simulink model "CPG_online"  (R2021b)
settings: Solver=FixedStepDiscrete  StartTime=0.0  StopTime=inf  FixedStep=Ts_cal  MaxStep=0.05  RelTol=0.5  AbsTol=0.5
model workspace (MATLAB code in the model file):
  | %---------------Critical values---------------%
  | angle_amp = pi/4; % Motor rotate amplitude, ref: pi/4
  | rotateCorrectionCoef = 1.158;
  | criticalFn = 2;
  | 
  | %------values for normalization---------------%
  | % values got by running manual gait
  | rotxNormGain = 1/0.1;
  | rotyNormGain = 1/0.05;
  | rotzNormGain = 1/0.1;
  | 
  | vxNormGain = 1/0.2;
  | vyNormGain = 1/0.2;
  | vzNormGain = 1/0.2;
  | 
  | FnNormGain = 1/15;
  | 
  | %--------values for check done---------------%
  | rotDone = pi/6;
  | legBendDone = pi/3; % actuator max bending angle
  | 
  | %---------------Robot parameters-------------%
  | % robot size
  | robot_width = 0.15;
  | robot_length = 0.22;
  | 
  | % floor parameters
  | floor_length = 2;
  | floor_width = 2;
  | 
  | % continuum actuator size
  | L_disk = 0.02944;% Disk side length (m)
  | R_w = L_disk/sqrt(3);
  | thickness_disk = 0.004; % Disk thickness (m)
  | thigh_length = 0.06;
  | R_core = 0.005; % Core radius (m)
  | length_core = 0.008; % Core length (m)
  | R_spool = 0.021; % 0.01944; % radius of the spool
  | spool_height = 0.022+0.015;
  | R_pulley = 1e-3;
  | spool_k = 0;
  | spool_d = 0;
  | hole_d = 4e-3;
  | 
  | % Material property
  | rho_PLA = 1.24e3;
  | rho = 1.19e3; % 1.19e3; % Density (kg/m^3)
  | % use rigid joints
  | Pz_stiff = 135000;
  | Pz_damping = 500;
  | S_stiff = 0.0239;
  | S_damping = 7.5e-5;
  | S_low_Bound = -20;
  | S_up_Bound = 20;
  | 
  | R_foot = 0.015; % foot radius (m)
  | 
  | % motor parameter
  | stall_T = 11.2/10; % 11.2 cm*kg, stall torque
  | t_60_deg = 0.2; % 0.09 s
  | V_nomrmal = 6; % corresponding normal voltage
  | Jr = 0.0001; %g*cm^2, robot inertia
  | 
  | % contact force
  | coef_static_friction = 0.315;
  | coef_dynamic_friction = 0.3;
  | crictic_velocity = 0.3; % m/s
  | contact_suf_stiff = 1000; % N/m
  | contact_suf_damp = 50; % N/(m/s)
  | contact_region_width = 2e-3; % m
  | spoolOpacity = 0;
  | tendonColor = [0.902 0.902 0.902];
  | tendonOpacity = 0.1;
  | 
  | % If use point masses
  | MMainFrame = 198; % g
  | MServoMotor = 50.55;
  | MMotorSupport = 12.1;
  | MSpool = 9.2;
  | 
  | % Robot total weight about 2 kg
  | MComposateLoad = 200;
  | 
  | MBuck = 40; % x2
  | MPCB_RPi = 141.3;
  | MLiBattery = 120; % x2
  | MPowerBank = 66.5;
  | isLoadVisible = 0.1;
  | 
  | 
  | MThigh = 26.7963;
  | MCore = 0.747699;
  | MDisk = 1.78642;
  | MFoot = 16.8232;
values from neighbouring files (symbols this model uses):
  A = [0 Ts; 0 1]    [MFBO_main.m]    (also in MFGP_main.m)
  A_cpg = 1    [MFBO_main.m]    (also in MFGP_main.m)
  alpha = opt_param(2)    [MFBO_main.m]    (also in MFGP_main.m)
  alpha_b_gain = opt_param(3)    [MFBO_main.m]    (also in MFGP_main.m)
  alpha_r_gain = pi    (= 3.14159265359)    [MFBO_main.m]    (also in MFGP_main.m)
  B = [0.5*Ts^2; Ts]    [MFBO_main.m]    (also in MFGP_main.m)
  C = [1 0]    [MFBO_main.m]    (also in MFGP_main.m)
  epsilon = 5    [MFBO_main.m]    (also in MFGP_main.m)
  f = 1/T    [MFBO_main.m]    (also in MFGP_main.m)
  init_state = rand(1, 8)*2 - 1    [MFBO_main.m]    (also in MFGP_main.m)
  k = 1000    [MFBO_main.m]    (also in MFGP_main.m)
  phi_vec = pi*[-1; 1; -1; 1]    [MFBO_main.m]    (also in MFGP_main.m)
  R = 0.15    [MFBO_main.m]    (also in MFGP_main.m)
  tau = 1    [MFBO_main.m]    (also in MFGP_main.m)
  Ts = 5e-2    (= 0.05)    [MFBO_main.m]    (also in MFGP_main.m)
  Ts_cal = 5e-4    (= 0.0005)    [MFBO_main.m]    (also in MFGP_main.m)
  z_l_diff = opt_param(5)    [MFBO_main.m]    (also in MFGP_main.m)
  z_l_gain = opt_param(4)    [MFBO_main.m]    (also in MFGP_main.m)
undefined symbols (not defined in the file or in its folder): DiscIntNeverNeededParam, Discrete, Time
libraries: svdutilitieslib x15, simulink x4, ctrlSharedLib x3, instrumentlib x2, aerolibanimutils x1
(part 2 of 2)

== system CPG_online/Sensing/vy_cal ==
  left : Inport
  right : Inport  Port=2
  acc_y : Inport  Port=3
  Add : Sum  Inputs=+-
  Add1 : Sum  Inputs=+-
  Data Type Conversion1 : DataTypeConversion  OutDataTypeStr=double
  Data Type Conversion10 : DataTypeConversion  OutDataTypeStr=double
  Data Type Conversion9 : DataTypeConversion  OutDataTypeStr=double
  Delay : Delay  SampleTime=Ts
  Delay1 : Delay  DelayLength=1  SampleTime=Ts
  Delay2 : Delay  DelayLength=1  SampleTime=Ts
  Delay3 : Delay  DelayLength=1  SampleTime=Ts
  Gain : Gain  Gain=1/1000
  Gain12 : Gain  Gain=-1
  Kalman Filter : ctrlSharedLib/Kalman Filter  TimeDomain=Discrete-Time  UseCurrentEstimator=on  ModelSource=Individual A, B, C, D matrices  ModelSourceVariable=ss(0.95,1,1,0,1)  A=A  B=B  C=C  D=0  NumberOfStates=1  NumberOfInputs=1  NumberOfOutputs=1  InitialEstimateSource=Dialog  X0=[0;0]  P0=10  UseK=off  UseGH=off  NumberOfProcessNoiseInputs=1  G=1  TimeInvariantG=on  H=0  TimeInvariantH=on  Q=Q  TimeInvariantQ=on  R=R  TimeInvariantR=on  N=0  TimeInvariantN=on  AddInputPort=on  AddEnablePort=off  OutputEstimatedY=off  OutputP=off  Ts=Ts
  MATLAB Function : MATLAB Function  TreatAsAtomicUnit=on
  MATLAB Function1 : MATLAB Function  TreatAsAtomicUnit=on
  MATLAB Function2 : MATLAB Function  TreatAsAtomicUnit=on
  Terminator : Terminator
  vy : Outport
  wires:
  Delay1/1 -> MATLAB Function1/3(predd_acc)
  Delay/1 -> MATLAB Function1/2(pred_acc), Delay1/1
  acc_y/1 -> Data Type Conversion1/1
  MATLAB Function1/1(acceleration) -> Kalman Filter/1  "acc"
  Delay3/1 -> Add1/2
  Gain12/1 -> MATLAB Function/1(v_left)
  Data Type Conversion10/1 -> Delay2/1, Add/1  "v_left"
  right/1 -> Data Type Conversion10/1
  MATLAB Function/1(vy) -> Gain/1  "vy"
  left/1 -> Data Type Conversion9/1
  Data Type Conversion9/1 -> Add1/1, Delay3/1  "v_left"
  Gain/1 -> Kalman Filter/2  "vy"
  Delay2/1 -> Add/2
  Add/1 -> MATLAB Function/2(v_right)
  Add1/1 -> Gain12/1
  Data Type Conversion1/1 -> Delay/1, MATLAB Function1/1("acceleration ")
  Kalman Filter/1 -> MATLAB Function2/1(u)  "vy"
  MATLAB Function2/1(y) -> Terminator/1
  MATLAB Function2/2(v) -> vy/1

== system CPG_online/Sensing/vz_cal ==
  down : Inport
  acc_z : Inport  Port=2
  Add1 : Sum  Inputs=+-
  Data Type Conversion1 : DataTypeConversion  OutDataTypeStr=double
  Data Type Conversion9 : DataTypeConversion  OutDataTypeStr=double
  Delay : Delay  SampleTime=Ts
  Delay1 : Delay  DelayLength=1  SampleTime=Ts
  Delay3 : Delay  DelayLength=1  SampleTime=Ts
  Gain : Gain  Gain=1/1000
  Gain12 : Gain  Gain=-1
  Kalman Filter : ctrlSharedLib/Kalman Filter  TimeDomain=Discrete-Time  UseCurrentEstimator=on  ModelSource=Individual A, B, C, D matrices  ModelSourceVariable=ss(0.95,1,1,0,1)  A=A  B=B  C=C  D=0  NumberOfStates=1  NumberOfInputs=1  NumberOfOutputs=1  InitialEstimateSource=Dialog  X0=[0;0]  P0=10  UseK=off  UseGH=off  NumberOfProcessNoiseInputs=1  G=1  TimeInvariantG=on  H=0  TimeInvariantH=on  Q=Q  TimeInvariantQ=on  R=R  TimeInvariantR=on  N=0  TimeInvariantN=on  AddInputPort=on  AddEnablePort=off  OutputEstimatedY=off  OutputP=off  Ts=Ts
  MATLAB Function : MATLAB Function  TreatAsAtomicUnit=on
  MATLAB Function1 : MATLAB Function  TreatAsAtomicUnit=on
  MATLAB Function2 : MATLAB Function  TreatAsAtomicUnit=on
  Terminator : Terminator
  vz : Outport
  wires:
  Delay1/1 -> MATLAB Function1/3(predd_acc)
  Delay/1 -> MATLAB Function1/2(pred_acc), Delay1/1
  acc_z/1 -> Data Type Conversion1/1
  MATLAB Function1/1(acceleration) -> Kalman Filter/1  "acc"
  Delay3/1 -> Add1/2
  Gain12/1 -> MATLAB Function/1(v_down)
  MATLAB Function/1(vz) -> Gain/1  "vz"
  down/1 -> Data Type Conversion9/1
  Data Type Conversion9/1 -> Add1/1, Delay3/1
  Gain/1 -> Kalman Filter/2  "vz"
  Add1/1 -> Gain12/1  "v_down"
  Data Type Conversion1/1 -> Delay/1, MATLAB Function1/1("acceleration ")
  Kalman Filter/1 -> MATLAB Function2/1(u)  "vz"
  MATLAB Function2/2(v) -> vz/1
  MATLAB Function2/1(y) -> Terminator/1

== system CPG_online/Subsystem/FL ==
  act : Inport
  Add : Sum
  Constant : Constant
  Demux1 : Demux  Outputs=3
  Gain : Gain  Gain=alpha_r_gain
  Gain1 : Gain  Gain=alpha_b_gain
  Gain2 : Gain  Gain=z_l_gain/2
  MATLAB Function : MATLAB Function  TreatAsAtomicUnit=on
  Mux3 : Mux  Inputs=3
  angle : Outport
  wires:
  MATLAB Function/3(alpha_C) -> Mux3/3
  Demux1/2 -> Gain1/1  "alpha_b_Ref"
  Gain1/1 -> MATLAB Function/2(alpha_b)
  Constant/1 -> Add/2
  MATLAB Function/1(alpha_A) -> Mux3/1
  MATLAB Function/2(alpha_B) -> Mux3/2
  Gain2/1 -> MATLAB Function/3(z_l)
  Demux1/3 -> Add/1  "z_l_Ref"
  Demux1/1 -> Gain/1  "alpha_r_Ref"
  Gain/1 -> MATLAB Function/1(alpha_r)
  Add/1 -> Gain2/1
  Mux3/1 -> angle/1
  act/1 -> Demux1/1

== system CPG_online/Subsystem/FR ==
  act : Inport
  Add : Sum
  Constant : Constant
  Demux1 : Demux  Outputs=3
  Gain : Gain  Gain=alpha_r_gain
  Gain1 : Gain  Gain=alpha_b_gain
  Gain2 : Gain  Gain=z_l_gain/2
  MATLAB Function : MATLAB Function  TreatAsAtomicUnit=on
  Mux3 : Mux  Inputs=3
  angle : Outport
  wires:
  MATLAB Function/3(alpha_C) -> Mux3/3
  Demux1/2 -> Gain1/1  "alpha_b_Ref"
  Gain1/1 -> MATLAB Function/2(alpha_b)
  Constant/1 -> Add/2
  MATLAB Function/1(alpha_A) -> Mux3/1
  MATLAB Function/2(alpha_B) -> Mux3/2
  Gain2/1 -> MATLAB Function/3(z_l)
  Demux1/3 -> Add/1  "z_l_Ref"
  Demux1/1 -> Gain/1  "alpha_r_Ref"
  Gain/1 -> MATLAB Function/1(alpha_r)
  Add/1 -> Gain2/1
  Mux3/1 -> angle/1
  act/1 -> Demux1/1

== system CPG_online/Subsystem/RL ==
  act : Inport
  Add : Sum
  Constant : Constant
  Demux1 : Demux  Outputs=3
  Gain : Gain  Gain=alpha_r_gain
  Gain1 : Gain  Gain=alpha_b_gain
  Gain2 : Gain  Gain=z_l_gain/2
  MATLAB Function : MATLAB Function  TreatAsAtomicUnit=on
  Mux3 : Mux  Inputs=3
  angle : Outport
  wires:
  MATLAB Function/3(alpha_C) -> Mux3/3
  Demux1/2 -> Gain1/1  "alpha_b_Ref"
  Gain1/1 -> MATLAB Function/2(alpha_b)
  Constant/1 -> Add/2
  MATLAB Function/1(alpha_A) -> Mux3/1
  MATLAB Function/2(alpha_B) -> Mux3/2
  Gain2/1 -> MATLAB Function/3(z_l)
  Demux1/3 -> Add/1  "z_l_Ref"
  Demux1/1 -> Gain/1  "alpha_r_Ref"
  Gain/1 -> MATLAB Function/1(alpha_r)
  Add/1 -> Gain2/1
  Mux3/1 -> angle/1
  act/1 -> Demux1/1

== system CPG_online/Subsystem/RR ==
  act : Inport
  Add : Sum
  Constant : Constant
  Demux1 : Demux  Outputs=3
  Gain : Gain  Gain=alpha_r_gain
  Gain1 : Gain  Gain=alpha_b_gain
  Gain2 : Gain  Gain=z_l_gain/2
  MATLAB Function : MATLAB Function  TreatAsAtomicUnit=on
  Mux3 : Mux  Inputs=3
  angle : Outport
  wires:
  MATLAB Function/3(alpha_C) -> Mux3/3
  Demux1/2 -> Gain1/1  "alpha_b_Ref"
  Gain1/1 -> MATLAB Function/2(alpha_b)
  Constant/1 -> Add/2
  MATLAB Function/1(alpha_A) -> Mux3/1
  MATLAB Function/2(alpha_B) -> Mux3/2
  Gain2/1 -> MATLAB Function/3(z_l)
  Demux1/3 -> Add/1  "z_l_Ref"
  Demux1/1 -> Gain/1  "alpha_r_Ref"
  Gain/1 -> MATLAB Function/1(alpha_r)
  Add/1 -> Gain2/1
  Mux3/1 -> angle/1
  act/1 -> Demux1/1

== system CPG_online/Sensing/rot_cal/Subsystem ==
  rotz_raw : Inport
  Abs : Abs
  Delay : Delay  DelayLength=1
  Subtract : Sum  Inputs=-+
  Switch : Switch  Criteria=u2 > Threshold  Threshold=0.2
  rotz : Outport
  wires:
  rotz_raw/1 -> Switch/3, Subtract/2
  Delay/1 -> Switch/1, Subtract/1
  Abs/1 -> Switch/2
  Subtract/1 -> Abs/1
  Switch/1 -> Delay/1, rotz/1

== system CPG_online/Sensing/rot_cal/Subsystem1 ==
  roty_raw : Inport
  Abs : Abs
  Delay : Delay  DelayLength=1
  Subtract : Sum  Inputs=-+
  Switch : Switch  Criteria=u2 > Threshold  Threshold=0.2
  roty : Outport
  wires:
  roty_raw/1 -> Switch/3, Subtract/2
  Delay/1 -> Switch/1, Subtract/1
  Abs/1 -> Switch/2
  Subtract/1 -> Abs/1
  Switch/1 -> Delay/1, roty/1

== system CPG_online/Sensing/rot_cal/Subsystem2 ==
  rotx_raw : Inport
  Abs : Abs
  Delay : Delay  DelayLength=1
  Subtract : Sum  Inputs=-+
  Switch : Switch  Criteria=u2 > Threshold  Threshold=0.2
  rotx : Outport
  wires:
  rotx_raw/1 -> Switch/3, Subtract/2
  Delay/1 -> Switch/1, Subtract/1
  Abs/1 -> Switch/2
  Subtract/1 -> Abs/1
  Switch/1 -> Delay/1, rotx/1

== matlab function CPG_online/Subsystem/RL/MATLAB Function ==
  data: alpha_r input; alpha_A output; alpha_b input; z_l input; alpha_B output; alpha_C output
function [alpha_A, alpha_B, alpha_C]= fcn(alpha_r, alpha_b, z_l)

L_disk = 0.02944;% Disk side length (m)
R_spool = 0.021;
R_w = L_disk/sqrt(3);

alpha_A = (-R_w*alpha_b*cos(-alpha_r)+z_l)/R_spool;
alpha_B = (-R_w*alpha_b*cos(-alpha_r+2*pi/3)+z_l)/R_spool;
alpha_C = (-R_w*alpha_b*cos(-alpha_r+4*pi/3)+z_l)/R_spool;

== matlab function CPG_online/CPG_cont/Hopf_oscillator (leg#2)/adaptive_f ==
  data: alpha input; f_a output; f input; tau input; v input
 % calculate the adaptive frequency f through (4) in 
 % 'Design and Locomotion Control of a Biomimetic Underwater Vehicle ... '
function f_a = adaptive_f(alpha, f, tau, v)
    f1 = f/2/alpha;
    f2 = (2*alpha - 1)*f/(2*alpha*(1 - alpha)*(1 + exp(-tau*v)));
    f_a = f1 + f2;

== matlab function CPG_online/CPG_cont/Hopf_oscillator (leg#3)/adaptive_f ==
  data: alpha input; f_a output; f input; tau input; v input
 % calculate the adaptive frequency f through (4) in 
 % 'Design and Locomotion Control of a Biomimetic Underwater Vehicle ... '
function f_a = adaptive_f(alpha, f, tau, v)
    f1 = f/2/alpha;
    f2 = (2*alpha - 1)*f/(2*alpha*(1 - alpha)*(1 + exp(-tau*v)));
    f_a = f1 + f2;

== matlab function CPG_online/Sensing/vy_cal/MATLAB Function ==
  data: v_left input; vy output; v_right input
function vy = fcn(v_left, v_right)

if abs(v_left) >= 20 && abs(v_right) < 20
    vy = v_right;
elseif abs(v_right) >= 20 && abs(v_left) < 20
    vy = v_left;
else
    vy = (v_right + v_left)/2;
end

== matlab function CPG_online/CPG_cont/Hopf_oscillator (leg#4)/adaptive_f ==
  data: alpha input; f_a output; f input; tau input; v input
 % calculate the adaptive frequency f through (4) in 
 % 'Design and Locomotion Control of a Biomimetic Underwater Vehicle ... '
function f_a = adaptive_f(alpha, f, tau, v)
    f1 = f/2/alpha;
    f2 = (2*alpha - 1)*f/(2*alpha*(1 - alpha)*(1 + exp(-tau*v)));
    f_a = f1 + f2;

== matlab function CPG_online/CPG_cont/leg_coupling ==
  data: epsilon input; u_vec input; C_leg1 output size=2; v_vec input; phi_vec input; C_leg2 output size=2; C_leg3 output size=2; C_leg4 output size=2
% epsilon: 1X1
% u_vec: 4X1
% v_vec: 4X1
% phi_vec: 4X1
% C_leg1-4 : 2X1
function [C_leg1, C_leg2, C_leg3, C_leg4] = fcn(epsilon, u_vec, v_vec, phi_vec)
    C1 = 0;
    % first leg
    C21 = epsilon*(-u_vec(4)*sin(phi_vec(4)) + v_vec(4)*cos(phi_vec(4)) - ...
                   -u_vec(1)*sin(phi_vec(1)) + v_vec(2)*cos(phi_vec(1)));
    C22 = epsilon*(-u_vec(1)*sin(phi_vec(1)) + v_vec(1)*cos(phi_vec(1)) - ...
                   -u_vec(2)*sin(phi_vec(2)) + v_vec(3)*cos(phi_vec(2)));
    C23 = epsilon*(-u_vec(2)*sin(phi_vec(2)) + v_vec(2)*cos(phi_vec(2)) - ...
                   -u_vec(3)*sin(phi_vec(3)) + v_vec(4)*cos(phi_vec(3)));
    C24 = epsilon*(-u_vec(3)*sin(phi_vec(3)) + v_vec(3)*cos(phi_vec(3)) - ...
                   -u_vec(4)*sin(phi_vec(4)) + v_vec(1)*cos(phi_vec(4)));
    
    C_leg1 = [C1; C21];
    C_leg2 = [C1; C22];
    C_leg3 = [C1; C23];
    C_leg4 = [C1; C24];

== matlab function CPG_online/CPG/Hopf_oscillator (leg#4)/adaptive_f ==
  data: alpha input; f_a output; f input; tau input; v input
 % calculate the adaptive frequency f through (4) in 
 % 'Design and Locomotion Control of a Biomimetic Underwater Vehicle ... '
function f_a = adaptive_f(alpha, f, tau, v)
    f1 = f/2/alpha;
    f2 = (2*alpha - 1)*f/(2*alpha*(1 - alpha)*(1 + exp(-tau*v)));
    f_a = f1 + f2;

== matlab function CPG_online/CPG/leg_coupling ==
  data: epsilon input; u_vec input; C_leg1 output size=2; v_vec input; phi_vec input; C_leg2 output size=2; C_leg3 output size=2; C_leg4 output size=2
% epsilon: 1X1
% u_vec: 4X1
% v_vec: 4X1
% phi_vec: 4X1
% C_leg1-4 : 2X1
function [C_leg1, C_leg2, C_leg3, C_leg4] = fcn(epsilon, u_vec, v_vec, phi_vec)
    C1 = 0;
    % first leg
    C21 = epsilon*(-u_vec(4)*sin(phi_vec(4)) + v_vec(4)*cos(phi_vec(4)) - ...
                   -u_vec(1)*sin(phi_vec(1)) + v_vec(2)*cos(phi_vec(1)));
    C22 = epsilon*(-u_vec(1)*sin(phi_vec(1)) + v_vec(1)*cos(phi_vec(1)) - ...
                   -u_vec(2)*sin(phi_vec(2)) + v_vec(3)*cos(phi_vec(2)));
    C23 = epsilon*(-u_vec(2)*sin(phi_vec(2)) + v_vec(2)*cos(phi_vec(2)) - ...
                   -u_vec(3)*sin(phi_vec(3)) + v_vec(4)*cos(phi_vec(3)));
    C24 = epsilon*(-u_vec(3)*sin(phi_vec(3)) + v_vec(3)*cos(phi_vec(3)) - ...
                   -u_vec(4)*sin(phi_vec(4)) + v_vec(1)*cos(phi_vec(4)));
    
    C_leg1 = [C1; C21];
    C_leg2 = [C1; C22];
    C_leg3 = [C1; C23];
    C_leg4 = [C1; C24];

== matlab function CPG_online/Sensing/vx_cal/MATLAB Function1 ==
  data: acceleration input; acceleration output; pred_acc input; predd_acc input
function acceleration = fcn(acceleration,pred_acc,predd_acc)
    if abs(acceleration) < 0.1
        acceleration = 0;
    end
    
    if abs(acceleration) > 10
        acceleration = (pred_acc+predd_acc)/2;
    end
end

== matlab function CPG_online/Sensing/vx_cal/MATLAB Function2 ==
  data: u input; y output; v output
function [y, v] = fcn(u)

y = u(1);
v = u(2);

== matlab function CPG_online/Sensing/vy_cal/MATLAB Function1 ==
  data: acceleration input; acceleration output; pred_acc input; predd_acc input
function acceleration = fcn(acceleration,pred_acc,predd_acc)
    if abs(acceleration) < 0.1
        acceleration = 0;
    end
    
    if abs(acceleration) > 10
        acceleration = (pred_acc+predd_acc)/2;
    end
end

== matlab function CPG_online/Sensing/vz_cal/MATLAB Function ==
  data: v_down input; vz output
function vz = fcn(v_down)

if v_down >= 20 
    vz = 20;
elseif v_down <= -20
    vz = -20;
else
    vz = v_down;
end

== matlab function CPG_online/CPG/Hopf_oscillator (leg#1)/adaptive_f ==
  data: alpha input; f_a output; f input; tau input; v input
 % calculate the adaptive frequency f through (4) in 
 % 'Design and Locomotion Control of a Biomimetic Underwater Vehicle ... '
function f_a = adaptive_f(alpha, f, tau, v)
    f1 = f/2/alpha;
    f2 = (2*alpha - 1)*f/(2*alpha*(1 - alpha)*(1 + exp(-tau*v)));
    f_a = f1 + f2;

== matlab function CPG_online/Sensing/vz_cal/MATLAB Function1 ==
  data: acceleration input; acceleration output; pred_acc input; predd_acc input
function acceleration = fcn(acceleration,pred_acc,predd_acc)
    if abs(acceleration) < 0.1
        acceleration = 0;
    end
    
    if abs(acceleration) > 10
        acceleration = (pred_acc+predd_acc)/2;
    end
end

== matlab function CPG_online/Sensing/vy_cal/MATLAB Function2 ==
  data: u input; y output; v output
function [y, v] = fcn(u)

y = u(1);
v = u(2);

== matlab function CPG_online/Sensing/vz_cal/MATLAB Function2 ==
  data: u input; y output; v output
function [y, v] = fcn(u)

y = u(1);
v = u(2);

== matlab function CPG_online/CPG/Hopf_oscillator (leg#2)/adaptive_f ==
  data: alpha input; f_a output; f input; tau input; v input
 % calculate the adaptive frequency f through (4) in 
 % 'Design and Locomotion Control of a Biomimetic Underwater Vehicle ... '
function f_a = adaptive_f(alpha, f, tau, v)
    f1 = f/2/alpha;
    f2 = (2*alpha - 1)*f/(2*alpha*(1 - alpha)*(1 + exp(-tau*v)));
    f_a = f1 + f2;

== matlab function CPG_online/Sensing/vx_cal/MATLAB Function ==
  data: v_front input; vx output; v_back input
function vx = fcn(v_front, v_back)

if abs(v_front) >= 20 && abs(v_back) < 20
    vx = v_back;
elseif abs(v_back) >= 20 && abs(v_front) < 20
    vx = v_front;
else
    vx = (v_back + v_front)/2;
end

== matlab function CPG_online/CPG/Hopf_oscillator (leg#3)/adaptive_f ==
  data: alpha input; f_a output; f input; tau input; v input
 % calculate the adaptive frequency f through (4) in 
 % 'Design and Locomotion Control of a Biomimetic Underwater Vehicle ... '
function f_a = adaptive_f(alpha, f, tau, v)
    f1 = f/2/alpha;
    f2 = (2*alpha - 1)*f/(2*alpha*(1 - alpha)*(1 + exp(-tau*v)));
    f_a = f1 + f2;

== matlab function CPG_online/CPG_cont/Hopf_oscillator (leg#1)/adaptive_f ==
  data: alpha input; f_a output; f input; tau input; v input
 % calculate the adaptive frequency f through (4) in 
 % 'Design and Locomotion Control of a Biomimetic Underwater Vehicle ... '
function f_a = adaptive_f(alpha, f, tau, v)
    f1 = f/2/alpha;
    f2 = (2*alpha - 1)*f/(2*alpha*(1 - alpha)*(1 + exp(-tau*v)));
    f_a = f1 + f2;

== matlab function CPG_online/Subsystem/FR/MATLAB Function ==
  data: alpha_r input; alpha_A output; alpha_b input; z_l input; alpha_B output; alpha_C output
function [alpha_A, alpha_B, alpha_C]= fcn(alpha_r, alpha_b, z_l)

L_disk = 0.02944;% Disk side length (m)
R_spool = 0.021;
R_w = L_disk/sqrt(3);

alpha_A = (-R_w*alpha_b*cos(-alpha_r)+z_l)/R_spool;
alpha_B = (-R_w*alpha_b*cos(-alpha_r+2*pi/3)+z_l)/R_spool;
alpha_C = (-R_w*alpha_b*cos(-alpha_r+4*pi/3)+z_l)/R_spool;

== matlab function CPG_online/Subsystem/FL/MATLAB Function ==
  data: alpha_r input; alpha_A output; alpha_b input; z_l input; alpha_B output; alpha_C output
function [alpha_A, alpha_B, alpha_C]= fcn(alpha_r, alpha_b, z_l)

L_disk = 0.02944;% Disk side length (m)
R_spool = 0.021;
R_w = L_disk/sqrt(3);

alpha_A = (-R_w*alpha_b*cos(-alpha_r)+z_l)/R_spool;
alpha_B = (-R_w*alpha_b*cos(-alpha_r+2*pi/3)+z_l)/R_spool;
alpha_C = (-R_w*alpha_b*cos(-alpha_r+4*pi/3)+z_l)/R_spool;

== matlab function CPG_online/Subsystem/RR/MATLAB Function ==
  data: alpha_r input; alpha_A output; alpha_b input; z_l input; alpha_B output; alpha_C output
function [alpha_A, alpha_B, alpha_C]= fcn(alpha_r, alpha_b, z_l)

L_disk = 0.02944;% Disk side length (m)
R_spool = 0.021;
R_w = L_disk/sqrt(3);

alpha_A = (-R_w*alpha_b*cos(-alpha_r)+z_l)/R_spool;
alpha_B = (-R_w*alpha_b*cos(-alpha_r+2*pi/3)+z_l)/R_spool;
alpha_C = (-R_w*alpha_b*cos(-alpha_r+4*pi/3)+z_l)/R_spool;
